simulink model "Panchito_Modelo_Matematico"  (R2026b)
settings: Solver=VariableStepAuto
settings Model: Creator=david  LastModifiedBy=david

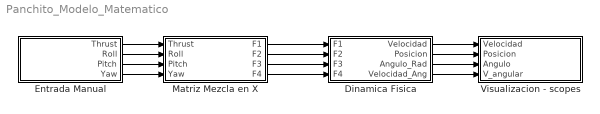
== system Panchito_Modelo_Matematico ==
  Dinamica Fisica : Subsystem
  Entrada Manual : Subsystem
  Matriz Mezcla en X : Subsystem
  Visualizacion - scopes : Subsystem
  wires:
  Entrada Manual/1(Thrust) -> Matriz Mezcla en X/1(Thrust)
  Entrada Manual/2(Roll) -> Matriz Mezcla en X/2(Roll)
  Entrada Manual/3(Pitch) -> Matriz Mezcla en X/3(Pitch)
  Entrada Manual/4(Yaw) -> Matriz Mezcla en X/4(Yaw)
  Matriz Mezcla en X/1(F1) -> Dinamica Fisica/1(F1)
  Matriz Mezcla en X/2(F2) -> Dinamica Fisica/2(F2)
  Matriz Mezcla en X/3(F3) -> Dinamica Fisica/3(F3)
  Matriz Mezcla en X/4(F4) -> Dinamica Fisica/4(F4)
  Dinamica Fisica/1(Velocidad) -> Visualizacion - scopes/1(Velocidad)
  Dinamica Fisica/2(Posicion) -> Visualizacion - scopes/2(Posicion)
  Dinamica Fisica/3(Angulo_Rad) -> Visualizacion - scopes/3(Angulo)
  Dinamica Fisica/4(Velocidad_Ang) -> Visualizacion - scopes/4(V_angular)

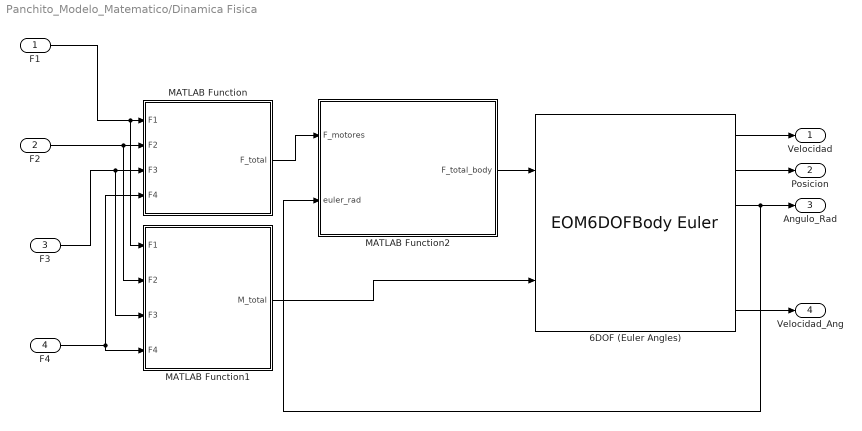
== system Panchito_Modelo_Matematico/Dinamica Fisica ==
  F1 : Inport
  F2 : Inport  Port=2
  F3 : Inport  Port=3
  F4 : Inport  Port=4
  6DOF (Euler Angles) : EOM6DOFBodyEuler  mass_0=0.0873
  MATLAB Function : MATLAB Function  TreatAsAtomicUnit=on
  MATLAB Function1 : MATLAB Function  TreatAsAtomicUnit=on
  MATLAB Function2 : MATLAB Function  TreatAsAtomicUnit=on
  Velocidad : Outport
  Posicion : Outport  Port=2
  Angulo_Rad : Outport  Port=3
  Velocidad_Ang : Outport  Port=4
  wires:
  6DOF (Euler Angles)/1 -> Velocidad/1
  6DOF (Euler Angles)/2 -> Posicion/1
  6DOF (Euler Angles)/3 -> MATLAB Function2/2(euler_rad), Angulo_Rad/1
  6DOF (Euler Angles)/6 -> Velocidad_Ang/1
  F1/1 -> MATLAB Function1/1(F1), MATLAB Function/1(F1)
  F2/1 -> MATLAB Function1/2(F2), MATLAB Function/2(F2)
  F3/1 -> MATLAB Function1/3(F3), MATLAB Function/3(F3)
  F4/1 -> MATLAB Function/4(F4), MATLAB Function1/4(F4)
  MATLAB Function1/1(M_total) -> 6DOF (Euler Angles)/2
  MATLAB Function/1(F_total) -> MATLAB Function2/1(F_motores)
  MATLAB Function2/1(F_total_body) -> 6DOF (Euler Angles)/1

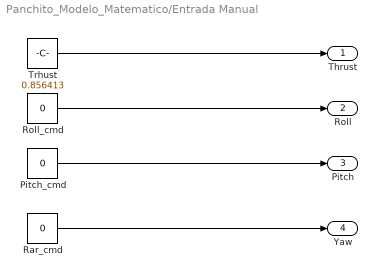
== system Panchito_Modelo_Matematico/Entrada Manual ==
  Pitch_cmd : Constant  Value=0
  Rar_cmd : Constant  Value=0
  Roll_cmd : Constant  Value=0
  Trhust : Constant  Value=0.856413
  Thrust : Outport
  Roll : Outport  Port=2
  Pitch : Outport  Port=3
  Yaw : Outport  Port=4
  wires:
  Trhust/1 -> Thrust/1
  Roll_cmd/1 -> Roll/1
  Pitch_cmd/1 -> Pitch/1
  Rar_cmd/1 -> Yaw/1

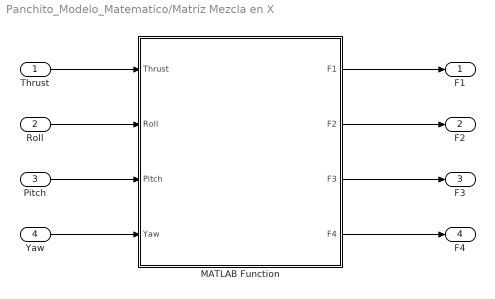
== system Panchito_Modelo_Matematico/Matriz Mezcla en X ==
  Thrust : Inport
  Roll : Inport  Port=2
  Pitch : Inport  Port=3
  Yaw : Inport  Port=4
  MATLAB Function : MATLAB Function  TreatAsAtomicUnit=on
  F1 : Outport
  F2 : Outport  Port=2
  F3 : Outport  Port=3
  F4 : Outport  Port=4
  wires:
  Thrust/1 -> MATLAB Function/1(Thrust)
  Roll/1 -> MATLAB Function/2(Roll)
  Pitch/1 -> MATLAB Function/3(Pitch)
  Yaw/1 -> MATLAB Function/4(Yaw)
  MATLAB Function/1(F1) -> F1/1
  MATLAB Function/2(F2) -> F2/1
  MATLAB Function/3(F3) -> F3/1
  MATLAB Function/4(F4) -> F4/1

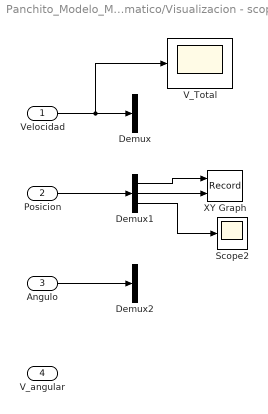
== system Panchito_Modelo_Matematico/Visualizacion - scopes ==
  Velocidad : Inport
  Posicion : Inport  Port=2
  Angulo : Inport  Port=3
  V_angular : Inport  Port=4
  Demux : Demux  Outputs=3
  Demux1 : Demux  Outputs=3
  Demux2 : Demux  Outputs=3
  Scope2 : Scope
      settings: ActiveDisplayYMinimum=-118.973547226542  ActiveDisplayYMaximum=667.68317245735989  DataLoggingVariableName=ScopeData3
  V_Total : Scope
      settings: ActiveDisplayYMinimum=-49.741077381253149  ActiveDisplayYMaximum=77.792520705717834
  XY Graph : Record  NumPorts=2.0  FileSettingsInternal="{\"entries\":[{\"content\":{\"excelSettings\":{\"content\":{},\"type\":\"Streamout.ExcelSettings\"},\"parquetSettings\":{\"content\":{},\"type\":\"Streamout.ParquetSettings\"}},\"type\":\"Streamout.FileSettingStorage\",\"uuid\":\"\"}],\"packageUris\":[\"http:\\/\\/schema.mathworks.com\\/mf0\\/streamout_blocks\\/R2020a\"],\"version\":\"1.0\"}"  FrameSettings=[0, 0]  Layout=[1 1]  SignalsInternal="{\"entries\":[{\"content\":{\"signals\":[{\"content\":{\"blockPath\":[],\"dimensions\":[1],\"domain\":\"\",\"lineColor\":\"#a2142f\",\"plots\":[ 1 ],\"port\":1,\"sid\":[\"\"],\"signalID\":1,\"signalName\":\"Demux1:1\"},\"type\":\"RecordBlkView.Signal\",\"uuid\":\"\"},{\"content\":{\"blockPath\":[],\"dimensions\":[1],\"domain\":\"\",\"lineColor\":\"#139fff\",\"plots\":[ 1 ],\"port\":2,\"sid\":[\"\"],\"signalID\":2,\"signalName\":\"Demux1:2\"},\"type\":\"RecordBlkView.Signal\",\"uuid\":\"\"}]},\"type\":\"RecordBlkView.InputSignals\",\"uuid\":\"\"}],\"packageUris\":[\"http:\\/\\/schema.mathworks.com\\/mf0\\/streamout_blocks\\/R2020a\"],\"version\":\"1.0\"}"  VisualizationBindings="{\"xyplotplugin\":{\"info\":[{\"series\":[{\"bindingParametersList\":[{\"parameter\":\"X-Axis\",\"signalID\":1,\"signalName\":\"Demux1:1\"},{\"parameter\":\"Y-Axis\",\"signalID\":2,\"signalName\":\"Demux1:2\"}],\"seriesID\":0}],\"subplotID\":1}]}}"  CompatibilityTag=XY
  wires:
  Velocidad/1 -> V_Total/1, Demux/1
  Posicion/1 -> Demux1/1
  Demux1/3 -> Scope2/1
  Angulo/1 -> Demux2/1
  Demux1/1 -> XY Graph/1
  Demux1/2 -> XY Graph/2

== matlab function Panchito_Modelo_Matematico/Dinamica Fisica/MATLAB Function ==
  data: F_total output; F1 input; F2 input; F3 input; F4 input
function F_total = calcular_fuerzas(F1, F2, F3, F4)
% Esta función recibe las 4 fuerzas individuales de los motores
% y regresa un vector columna de 3x1 con las fuerzas en los ejes X, Y, Z.

% 1. Inicializamos los componentes del vector
Fx = 0.0;
Fy = 0.0;

% 2. Sumamos las 4 fuerzas en el eje Z (Empuje vertical del dron)
Fz = F1 + F2 + F3 + F4;

% 3. Empaquetamos todo en un vector columna de 3x1 [X; Y; Z]
F_total = [Fx; Fy; Fz];
end

== matlab function Panchito_Modelo_Matematico/Matriz Mezcla en X/MATLAB Function ==
  data: Thrust input; F1 output; Roll input; Pitch input; Yaw input; F2 output; F3 output; F4 output
function [F1, F2, F3, F4] = mezcla_X(Thrust, Roll, Pitch, Yaw)
% lx y ly reales en metros para tu dron de 17x20 cm:
lx = 0.085;   % Distancia desde el centro al motor en el eje X (17cm / 2)
ly = 0.100;   % Distancia desde el centro al motor en el eje Y (20cm / 2)
gamma = 0.02; % Factor de torque de arrastre de la hélice

% Matriz de mezcla inversa calibrada para la geometría rectangular en X
% F1: Front Right (FR)
F1 = 0.25*Thrust + (1/(4*ly))*Roll + (1/(4*lx))*Pitch + (1/(4*gamma))*Yaw;
% F2: Front Left (FL)
F2 = 0.25*Thrust - (1/(4*ly))*Roll + (1/(4*lx))*Pitch - (1/(4*gamma))*Yaw;
% F3: Back Left (BL)
F3 = 0.25*Thrust - (1/(4*ly))*Roll - (1/(4*lx))*Pitch + (1/(4*gamma))*Yaw;
% F4: Back Right (BR)
F4 = 0.25*Thrust + (1/(4*ly))*Roll - (1/(4*lx))*Pitch - (1/(4*gamma))*Yaw;
end

== matlab function Panchito_Modelo_Matematico/Dinamica Fisica/MATLAB Function1 ==
  data: F1 input; M_total output; F2 input; F3 input; F4 input
function M_total = calcular_momentos(F1, F2, F3, F4)
% lx y ly reales en metros para tu dron de 17x20 cm:
lx = 0.085;   % Distancia desde el centro al motor en el eje X (17cm / 2)
ly = 0.100;   % Distancia desde el centro al motor en el eje Y (20cm / 2)
gamma = 0.02; % Factor de torque de arrastre de la hélice

% 1. Momento en X (Roll / Alabeo): Causado por la diferencia de fuerzas laterales
Mx = ly * (F1 - F2 - F3 + F4);

% 2. Momento en Y (Pitch / Cabeceo): Causado por la diferencia de fuerzas frontales/traseras
My = lx * (F1 + F2 - F3 - F4);

% 3. Momento en Z (Yaw / Guiñada): Causado por el torque de reacción aerodinámica de las hélices
Mz = gamma * (F1 - F2 + F3 - F4);

% 4. Empaquetamos todo en un vector columna de 3x1 [Mx; My; Mz]
M_total = [Mx; My; Mz];
end

== matlab function Panchito_Modelo_Matematico/Dinamica Fisica/MATLAB Function2 ==
  data: F_motores input; F_total_body output; euler_rad input
function F_total_body = entorno_dinamico(F_motores, euler_rad)
% F_motores: Vector 3x1 de tus motores [0; 0; F1+F2+F3+F4]
% euler_rad: Vector 3x1 que viene directo de la salida del 6 DOF [roll; pitch; yaw]

% 1. Datos físicos del dron
m = 0.0873; 
g = 9.81;

% 2. Separar los ángulos de inclinación actuales
phi   = euler_rad(1); % Roll
theta = euler_rad(2); % Pitch
% El Yaw (psi) no afecta la gravedad porque es giro sobre el eje vertical

% 3. Matriz de Rotación de la Tierra al Cuerpo (Trigonometría Aeroespacial)
% Esto calcula cómo ve el dron a la gravedad según qué tan inclinado esté
g_bx = -g * sin(theta);
g_by =  g * sin(phi) * cos(theta);
g_bz =  g * cos(phi) * cos(theta);

% 4. Vector de Fuerza de Gravedad en los ejes del dron (Peso dinámico)
W_body = [m * g_bx; 
    m * g_by; 
    m * g_bz];

% 5. Sumatoria final de fuerzas en los ejes del cuerpo (F_motores - Peso)
% Nota: El bloque 6 DOF toma el eje Z hacia ABAJO por estándar MKS aeronáutico.
% Por lo tanto, las hélices empujan en -Z y la gravedad jala en +Z.

Fx_total = F_motores(1) + W_body(1);
Fy_total = F_motores(2) + W_body(2);
Fz_total = -F_motores(3) + W_body(3); % Invierte el empuje hacia arriba

F_total_body = [Fx_total; Fy_total; Fz_total];
end
